simulink model "Flight_Controllers"  (R2024a)
settings: Solver=VariableStepAuto  StartTime=0.0  StopTime=tFinal  FixedStep=0.02  RelTol=1e-3
values from neighbouring files (symbols this model uses):
  bOmega = -bThrust/mThrust    (= 168.963839792)    [Load_VehicleParams.m]
  Cant_cosine_Loss = cos(fanCantAngle)    [Load_VehicleParams.m]
  g = 9.807    [Load_VehicleParams.m]
  g_Offset = 5/6    (= 0.833333333333)    [Load_VehicleParams.m]
  Kd_LatPos = 0    [Load_Controller_Gains_14.m]
  Kd_LatVel = 0    [Load_Controller_Gains_14.m]
  Kd_Pitch = 41.5    [Load_Controller_Gains_14.m]
  Ki_LatPos = 0    [Load_Controller_Gains_14.m]
  Ki_LatVel = 0    [Load_Controller_Gains_14.m]
  Ki_Pitch = 0.65    [Load_Controller_Gains_14.m]
  Kp_LatPos = 0.4    [Load_Controller_Gains_14.m]
  Kp_LatVel = -0.3    [Load_Controller_Gains_14.m]
  Kp_Pitch = 16    [Load_Controller_Gains_14.m]
  mOmega = 1/mThrust    (= 1.62153397114)    [Load_VehicleParams.m]
  N_LatPos = 0    [Load_Controller_Gains_14.m]
  N_LatVel = 0    [Load_Controller_Gains_14.m]
  N_Pitch = 85.6    [Load_Controller_Gains_14.m]
  nFans = 4    [Load_VehicleParams.m]
  pitch_Cmd_Limit = 7*pi/180    (= 0.12217304764)    [Load_Controller_Gains_14.m]
  tau_vCmd = 0.1    [Load_Controller_Gains_14.m]
  Ts_Control = 1/50    (= 0.02)    [run_Lander_GNC_Sim.m]
  velCmd_Limit = 7*pi/180    (= 0.12217304764)    [Load_Controller_Gains_14.m]
undefined symbols (not defined in the file or in its folder): den_Gc_z_Pitch, den_Gc_z_Pos, num_Gc_z_Pitch, num_Gc_z_Pos, posCntrl_Integr_Limit, tau_LatPos, tau_xCmd, vCmd_Integr_Limit
libraries: slpidlib x17
(part 3 of 3)

== matlab function Flight_Controllers/Lateral_Controllers/Lateral_Control_4/Lateral_Flight_Plan ==
  data: xCmd output; t input; LatFlt_Schedule input

function xCmd  = Lateral_Schedule(t, LatFlt_Schedule)

%  For Controller version 4 there is only 1 Lateral Control Mode and that is
%    Position Control.  Velocity is "controlled" indirectly by how the
%    position command is structured.
%  The Lateral Flight Schedule is arranged as follows:
%        Column 1:  Time (sec)
%        Column 2:  Mode   Always Mode 2 for Position Control
%        Column 3:  xCmd   X Position Command
%        Column 4:  vLim   Currently NOT used

% validateattributes(t, {'double'}, {'scalar'})

xCmd  = interp1( LatFlt_Schedule(:,1), LatFlt_Schedule(:,3), t); 
% vLim  = interp1( LatFlt_Schedule(:,1), LatFlt_Schedule(:,4), t, 'previous'); 

% modeLat = 2; %  Always Postion Mode.  Keeping this so the plot script is 
             %     good for this and Control schemes with more than one
             %     mode.

== matlab function Flight_Controllers/Lateral_Controllers/Lateral_Control_13/Lateral_Flight_Plan ==
  data: xCmd output; t input; LatFlt_Schedule input
function xCmd  = Lateral_Schedule(t, LatFlt_Schedule)

%  For Controller version 3 there is only 1 Lateral Control Mode and that is
%    Position Control.  Velocity is "controlled" indirectly by how the
%    position command is structured.
%  The Lateral Flight Schedule is arranged as follows:
%        Column 1:  Time (sec)
%        Column 2:  Mode   Always Mode 2 for Position Control
%        Column 3:  xCmd   X Position Command
%        Column 4:  vLim   Currently NOT used

% validateattributes(t, {'double'}, {'scalar'})

xCmd  = interp1( LatFlt_Schedule(:,1), LatFlt_Schedule(:,3), t); 
% vLim  = interp1( LatFlt_Schedule(:,1), LatFlt_Schedule(:,4), t, 'previous'); 

% modeLat = 2; %  Always Postion Mode.  Keeping this so the plot script is 
             %     good for this and Control schemes with more than one
             %     mode.

== matlab function Flight_Controllers/Lateral_Controllers/Lateral_Control_2/Lateral_Flight_Plan ==
  data: modeLat output; xCmd output; t input; vLim output; LatFlt_Schedule input
function [modeLat, xCmd, vLim] = Lateral_Schedule(t, LatFlt_Schedule)

%  For Controller version 2 there is only 1 Lateral Control Mode and that is
%    Position Control.  Velocity is "controlled" by a LIMIT on the
%    veloctity command coming from the Position Controller
%  The Lateral Flight Schedule is arranged as follows:
%        Column 1:  Time (sec)
%        Column 2:  Mode   Mode 1 is Velocity Control,  Mode 2 is Position Control
%        Column 3:  xCmd   X velocity command if in mode 1,  Position if in mode 2
%        Column 4:  vLim   X Velocity Limit

% validateattributes(t, {'double'}, {'scalar'})

xCmd  = interp1( LatFlt_Schedule(:,1), LatFlt_Schedule(:,3), t, 'previous'); 
vLim  = interp1( LatFlt_Schedule(:,1), LatFlt_Schedule(:,4), t, 'previous'); 

modeLat = 2; %  Always Postion Mode.  Keeping this so the plot script is 
             %     good for this and Control schemes with more than one
             %     mode.

== matlab function Flight_Controllers/Lateral_Controllers/Lateral_Control_1/Lateral_Flight_Plan ==
  data: t input; modeLat output; LatFlt_Schedule input; xCmd output; yCmd output
function [modeLat, xCmd, yCmd] = Lateral_Schedule(t, LatFlt_Schedule)

%  There are 2 Lateral Control Modes:  Velocity and Position
%  The Lateral Flight Schedule is arranged as follows:
%        Column 1:  Time (sec)
%        Column 2:  Mode   Mode 1 is Velocity Control,  Mode 2 is Position Control
%        Column 3:  xCmd   X velocity command if in mode 1,  Position if in mode 2
%        Column 4:  yCmd   Y velocity command if in mode 1,  Position if in mode 2

% validateattributes(t, {'double'}, {'scalar'})


modeLat = interp1( LatFlt_Schedule(:,1), LatFlt_Schedule(:,2), t, 'previous');
xCmd  = interp1( LatFlt_Schedule(:,1), LatFlt_Schedule(:,3), t, 'previous'); 
yCmd  = interp1( LatFlt_Schedule(:,1), LatFlt_Schedule(:,4), t, 'previous');

== matlab function Flight_Controllers/Lateral_Controllers/Lateral_Control_1/MATLAB Function ==
  data: Lat_Mode input; Vel_on_off output; Pos_on_off output
function [Vel_on_off, Pos_on_off] = fcn(Lat_Mode)

%   Mode 1 is Lateral Velocity Control,  Mode 2 is Lateral Position Control

if Lat_Mode > 1.5   %  Turn Position ON and Velocity OFF
    Vel_on_off = -1;  % Negative so Enabled System for velocity doesn't run
    Pos_on_off = 1;
else                   %  Turn Velocity ON and Positio OFF
    Vel_on_off =  1;  
    Pos_on_off = -1;  % Negative so Enabled System for position doesn't run
end

== matlab function Flight_Controllers/Lateral_Controllers/Lateral_Control_14/Lateral_Flight_Plan ==
  data: xCmd output; t input; LatFlt_Schedule input

function xCmd  = Lateral_Schedule(t, LatFlt_Schedule)

%  For Controller version 4 there is only 1 Lateral Control Mode and that is
%    Position Control.  Velocity is "controlled" indirectly by how the
%    position command is structured.
%  The Lateral Flight Schedule is arranged as follows:
%        Column 1:  Time (sec)
%        Column 2:  Mode   Always Mode 2 for Position Control
%        Column 3:  xCmd   X Position Command
%        Column 4:  vLim   Currently NOT used

% validateattributes(t, {'double'}, {'scalar'})

xCmd  = interp1( LatFlt_Schedule(:,1), LatFlt_Schedule(:,3), t); 
% vLim  = interp1( LatFlt_Schedule(:,1), LatFlt_Schedule(:,4), t, 'previous'); 

% modeLat = 2; %  Always Postion Mode.  Keeping this so the plot script is 
             %     good for this and Control schemes with more than one
             %     mode.
